simulink model "Experiment_0121_cs"  (R2019a)
settings: Solver=ode5  StartTime=0.0  StopTime=30  FixedStep=1/20  RelTol=1e-3
PreLoadFcn:
  | mbxruntime.callbacks.PreLoadFcn(bdroot);
PostLoadFcn:
  | mbxruntime.callbacks.PostLoadFcn(bdroot);
InitFcn:
  | mbxruntime.callbacks.InitFcn(bdroot);
StartFcn:
  | mbxruntime.callbacks.StartFcn(bdroot);
StopFcn:
  | mbxruntime.callbacks.StopFcn(bdroot);
model workspace (MAT data in the model file):
  mbox_table : struct (value not decoded)
  model_closed = 0
  sim_status = 0
undefined symbols (not defined in the file or in its folder): DiscIntNeverNeededParam, warningInitialVelocity, x0
libraries: simulink x37, PreScanSimulinkLibrary x16, simulink_extras x10, PreScanUsefulBlocks x1
(part 1 of 6)
CloseFcn:
  | mbxruntime.callbacks.CloseFcn(bdroot);
settings Model: Creator=PRESCAN  LastModifiedBy=HP
settings DataIOCC: LimitDataPoints=on  SaveFormat=Array  SignalLoggingSaveFormat=ModelDataLogs  ReturnWorkspaceOutputs=off
settings OptimizationCC: ExpressionDepthLimit=2147483647  InitFltsAndDblsToZero=on  LifeSpan=inf
settings DebuggingCC: SaveWithParameterizedLinksMsg=none  UnderspecifiedInitializationDetection=Classic  MergeDetectMultiDrivingBlocksExec=none  SignalResolutionControl=TryResolveAllWithWarning  MultiTaskDSMMsg=warning  MultiTaskCondExecSysMsg=none  FcnCallInpInsideContextMsg=warning  StateNameClashWarn=warning  SFUnexpectedBacktrackingDiag=warning  SFNoUnconditionalDefaultTransitionDiag=warning  SFExecutionAtInitializationDiag=none  ArithmeticOperatorsInVariantConditions=warning
settings HardwareCC: ProdBitPerPointer=32  ProdBitPerSizeT=32  ProdBitPerPtrDiffT=32  ProdLargestAtomicFloat=None  ProdIntDivRoundTo=Undefined  ProdEndianess=Unspecified  ProdWordSize=32  ProdHWDeviceType=32-bit Generic
settings ModelReferenceCC: UpdateModelReferenceTargets=IfOutOfDate  PropagateSignalLabelsOutOfModel=off
settings SFSimCC: SimUseLocalCustomCode=off  SimParseCustomCode=off
settings SFSimCC: SimCustomHeaderCode=|
  | #include "prescan.h"
  | #include "prescan_platform.h"
settings RTWCC: RTWUseLocalCustomCode=off
settings CodeAppCC: StateflowObjectComments=on
settings GRTTargetCC: TargetFcnLib=ansi_tfl_tmw.mat  TargetLangStandard=C89/C90 (ANSI)  GeneratePreprocessorConditionals=Disable all  CombineOutputUpdateFcns=off  GRTInterface=on
settings ConfigComp: CovMetricSettings=dw  CovHtmlReporting=on  CovSaveCumulativeToWorkspaceVar=on  CovSaveSingleToWorkspaceVar=on  CovExternalEMLEnable=off

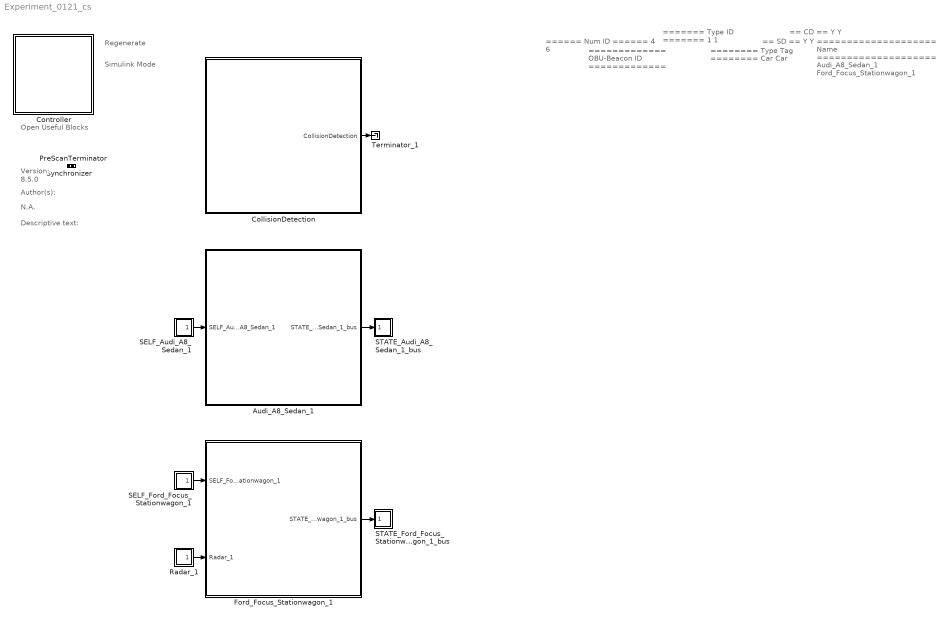
== system Experiment_0121_cs ==
  note: Regenerate
  note: Simulink Mode
  note: Open Useful Blocks
  note: 8.5.0
  note: Version:
  note: Author(s):
  note: N.A.
  note: Descriptive text:
  note: ======
      | Num ID
      | ======
      | 4
      | 6
  note: =============
      | OBU-Beacon ID
      | =============
  note: =======
      | Type ID
      | =======
      | 1
      | 1
  note: ========
      | Type Tag
      | ========
      | Car
      | Car
  note: ==
      | SD
      | ==
      | Y
      | Y
  note: ==
      | CD
      | ==
      | Y
      | Y
  note: ====================
      | Name
      | ====================
      | Audi_A8_Sedan_1
      | Ford_Focus_Stationwagon_1
  Audi_A8_Sedan_1 : Subsystem  Tag=WorldObjectSubSystem  InitFcn=UniqueId = '29';
      mask init:
      | modelPath = GenericModelHelper.getGenericModelFilePath('ModelDepo','Vehicles\Audi_A8\Audi_A8.pgmb','d771622804618130053427da08a6d484');imagePath = GenericModelHelper.getCompilationPicture(modelPath, 'Audi_A8_HighPoly.png');
      mask Display: image(imread(imagePath));color('white');text(0, 0, ' ID=4\n')
  CollisionDetection : Subsystem  Tag=sensor/CollisionDetection  Priority=3  LoadFcn=load('PrescanCollisionDetectionData.mat');load('PrescanCollisionDetectionMessage.mat')  mask(PreScan Source Block: CollisionDetection){}
      mask help: Collision Detection can be used to detect collisions between PreScan components. For Collision Detection the actual component shape is taken into account, so it is not a bounding box approach.
      settings: OpenFcn=open_system([gcb '/Sensor'],'mask')
      mask Help: eval('openHelp(811)')
      mask Display: image(imread('crash.jpg'))
  Controller : Subsystem  Description=35CC70460C0F6B9A74A5D35B42843DB509CCAA918CC068CE424F94149DBB7D73  Priority=-1  LoadFcn=load PreScanControllerData  mask(PreScan Simulation Controller){prescanversion='8.5.0', ModelReferencing=off, TimeStep=1/20, ControlMode=0, PreScanExecutionMode=on, ControllerCount=0, ControllerIndex=0, ControllerOptions=''}
      mask prompts: prescanversion "PreScan Version"; ModelReferencing "Use Model Referencing"; TimeStep "Upload Period [s]"; ControlMode "Control Mode"; PreScanExecutionMode "Execution Mode"; ControllerCount "Controller Count"; ControllerIndex "Controller Index"; ControllerOptions "Controller Options"
      mask help:
      | Please do not remove this block from the compilation sheet,
      | as it connects the model to the PreScan environment.
      mask init:
      | model = bdroot(gcb);
      | ExperimentFile = mbxruntime.findExperimentFile(model,true); %relative path
      | 
      | [d1, d2, d3, prescandata] = prescan_Settings();
      | ModelDepo = fullfile(prescandata,'ModelDepo'); 
      | 
      | RTmode = mbxruntime.getRTMode(model);
      | 
      | SimulationMode = get_param(bdroot,'SimulationMode');
      | if strcmp(SimulationMode, 'rapid-accelerator')
      |     SimulationMode = 'external';
      | end
      | TargetName = get_param(bdroot,'SystemTargetFile');
      settings: ModelCloseFcn=assignin('base',['model_closed_' bdroot],true);
      mask Help: eval('openHelp(812)')
      mask Display: image(imread('prescanlogo.ico'))
  Ford_Focus_Stationwagon_1 : Subsystem  Tag=WorldObjectSubSystem  InitFcn=UniqueId = '32';
      mask init:
      | modelPath = GenericModelHelper.getGenericModelFilePath('ModelDepo','Vehicles\Ford_Focus_Wagon\Ford_Focus_Wagon.pgmb','9f2f84850ce6f49365560c3439563633');imagePath = GenericModelHelper.getCompilationPicture(modelPath, 'Ford_Focus_Wagon_HighPoly.png');
      mask Display: image(imread(imagePath));color('white');text(0, 0, ' ID=6\n')
  PreScanTerminator : Subsystem  Tag=PreScanTerminator  Priority=999  LoadFcn=load PrescanTerminatorData  mask(PreScan Simulation Terminator){TimeStep=1/20}
      mask prompts: TimeStep "Upload Period [s]"
      mask help:
      | Please do not remove this block from the compilation sheet as it
      | connects the model to the PreScan environment.
      mask Help: eval('openHelp(812)')
      mask Display: image(imread('prescanlogo.ico'))
  Radar_1 : Subsystem  Tag=sensor/Radar  Priority=3  LoadFcn=load('PrescanScannerSensorData.mat');load('PrescanScannerSensorMessage.mat')  mask(PreScan Source Block: Radar Sensor){}
      mask help:
      | The Radar Sensor is a detailed sensor based on a physical radar
      | model that includes Antenna GAIN Maps (AGM) and atmospheric
      | attenuation.
      |
      | For more information, please click Help.
      settings: OpenFcn=open_system([gcb '/Sensor'],'mask')
      mask Help: eval('openHelp(1464)')
      mask Display: image(imread('Radar.png'))
  SELF_Audi_A8_Sedan_1 : Subsystem  Tag=sensor/SelfPort  Priority=3  LoadFcn=load('PreScanSelfSensorData.mat')  mask(PreScan Source Block: SELF){}
      mask help:
      | The SELF port shows (state) information of the actor itself. The outputs are position in the experiment's axis system and the GPS coordinates, and the object's absolute velocity and compass heading.
      |
      | For more information, please click Help.
      settings: OpenFcn=open_system([gcb '/Sensor'],'mask')
      mask Help: eval('openHelp(462)')
      mask Display: image(imread('GPS.png'))
  SELF_Ford_Focus_Stationwagon_1 : Subsystem  Tag=sensor/SelfPort  Priority=3  LoadFcn=load('PreScanSelfSensorData.mat')  mask(PreScan Source Block: SELF){}
      mask help:
      | The SELF port shows (state) information of the actor itself. The outputs are position in the experiment's axis system and the GPS coordinates, and the object's absolute velocity and compass heading.
      |
      | For more information, please click Help.
      settings: OpenFcn=open_system([gcb '/Sensor'],'mask')
      mask Help: eval('openHelp(462)')
      mask Display: image(imread('GPS.png'))
  STATE_Audi_A8_Sedan_1_bus : Subsystem  Tag=actuator/StatePort  Priority=0  LoadFcn=load('PreScanStateActuatorData.mat')  mask(PreScan Sink Block: State){}
      mask help:
      | The Actor State contains a vector signal of size (9x1), containing the following signals:
      |
      | -  Position    	(x,y,z)             	[m]
      | -  Velocity    	(vx,vy,vz)         	[m/s]
      | -  Angles       	(Roll, Pitch, Yaw)	[rad]
      |
      | The Actor state is defined in the global axis system.
      | The state is superponed on the Initial position defined in the GUI.
      |
      | For more information, please click Help.
      settings: OpenFcn=open_system([gcb '/Actuator'],'mask')
      mask Help: eval('openHelp(222)')
      mask Display: image(imread('State.png'))
  STATE_Ford_Focus_Stationwagon_1_bus : Subsystem  Tag=actuator/StatePort  Priority=0  LoadFcn=load('PreScanStateActuatorData.mat')  mask(PreScan Sink Block: State){}
      mask help:
      | The Actor State contains a vector signal of size (9x1), containing the following signals:
      |
      | -  Position    	(x,y,z)             	[m]
      | -  Velocity    	(vx,vy,vz)         	[m/s]
      | -  Angles       	(Roll, Pitch, Yaw)	[rad]
      |
      | The Actor state is defined in the global axis system.
      | The state is superponed on the Initial position defined in the GUI.
      |
      | For more information, please click Help.
      settings: OpenFcn=open_system([gcb '/Actuator'],'mask')
      mask Help: eval('openHelp(222)')
      mask Display: image(imread('State.png'))
  Synchronizer : Subsystem  Tag=PreScanSynchronizer  Priority=1  LoadFcn=load PrescanSynchronizeData  mask(PreScan Simulation Core Block){TimeStep=1/20}
      mask prompts: TimeStep "Timestep [s]"
      mask help:
      | Please do not remove this block from the PreScan compilation sheet,
      | as it contains essential configuration parameters for a PreScan simulation.
      settings: DeleteFcn=PreScanBlockDeleteFcn;
      mask Display: image(imread('prescanlogo.ico'))
  Terminator_1 : Terminator
  wires:
  Audi_A8_Sedan_1/1(STATE_Audi_A8_Sedan_1_bus) -> STATE_Audi_A8_Sedan_1_bus/1(STATE_Audi_A8_Sedan_1_bus)
  SELF_Audi_A8_Sedan_1/1(SELF_Audi_A8_Sedan_1) -> Audi_A8_Sedan_1/1(SELF_Audi_A8_Sedan_1)
  Ford_Focus_Stationwagon_1/1(STATE_Ford_Focus_Stationwagon_1_bus) -> STATE_Ford_Focus_Stationwagon_1_bus/1(STATE_Ford_Focus_Stationwagon_1_bus)
  SELF_Ford_Focus_Stationwagon_1/1(SELF_Ford_Focus_Stationwagon_1) -> Ford_Focus_Stationwagon_1/1(SELF_Ford_Focus_Stationwagon_1)
  Radar_1/1(Radar_1) -> Ford_Focus_Stationwagon_1/2(Radar_1)
  CollisionDetection/1(CollisionDetection) -> Terminator_1/1

== system Experiment_0121_cs/Audi_A8_Sedan_1 ==
  SELF_Audi_A8_Sedan_1 : Inport  Tag=inport/SelfPort  OutDataTypeStr=Bus: PRESCAN_SELFSENSORDATA  PortDimensions=1  SampleTime=1/20  BusOutputAsStruct=on
  Auto_Gear : Constant  Tag=AutoGear
  Dynamics_Simple : Subsystem  Tag=Simple_Vehicle_Dynamics  mask(PreScan Block: Simple Dynamics){Migrate=on, TimeStep=1/20, ComputationMode=Continuous_Time}
      mask prompts: Migrate "Migrate. During migration this block will be replaced by a newer one."; TimeStep "Auto assigned: Time Step [s]"; ComputationMode "Computation mode:"
      mask help:
      | The Simple Dynamics Model is selected in the GUI to simulate vehicle dynamics behavior.
      |
      | The Simple Dynamics Model is completely open to the user. The parameters of this model can be set in the Simple Dynamics dialog in the GUI.
      |
      | For more information, please click Help.
      mask init:
      | p = SimpleDyn_pars;
      settings: DeleteFcn=PreScanBlockDeleteFcn;
      mask Help: eval('openHelp(220)')
      mask Display:
      | image(imread('SimpleDyn.png'))
      | port_label('input', 1, '{\delta}_S_t_ _e_e_r [deg]','texmode','on')
      | port_label('input', 2, 'Throttle [%]')
      | port_label('input', 3, 'Brake Pres [bar]')
      | port_label('input', 4, 'V_0 [ms-1]','texmode','on')
      | port_label('input', 5, 'Auto=[0]/Manual=[1]')
      | port_label('input', 6, 'Auto_GearShift')
      | port_label('input', 7, 'Manual_GearShift')
      | port_label('output', 1, 'State')
      | port_label('output', 2, 'Vx [ms-1]')
      | port_label('output', 3, 'Perf Params')
  Ground_{1..6} (6 alike) : Ground
  SELF_Demux : Subsystem  Tag=demux/SelfPort  mask(PreScan Demux Block:){}
      mask help:
      | The SELF port shows (state) information of the actor itself. The outputs are position in the experiment's axis system and the GPS coordinates, and the object's absolute velocity and compass heading.
      |
      | For more information, please click Help.
      settings: DeleteFcn=PreScanBlockDeleteFcn;
      mask Help: eval('openHelp(462)')
      mask Display:
      | port_label('output',1,'x [m]')
      | port_label('output',2,'y [m]')
      | port_label('output',3,'z [m]','texmode','on')
      | port_label('output',4,'Rotx [deg]','texmode','on')
      | port_label('output',5,'Roty [deg]','texmode','on')
      | port_label('output',6,'Rotz [deg]','texmode','on')
      | port_label('output',7,'GPS lat [deg]','texmode','on')
      | port_label('output',8,'GPS long [deg]','texmode','on')
      | port_label('output',9,'GPS alt [m]','texmode','on')
      | port_label('output',10,'Velocity [m/s]')
      | port_label('output',11,'Heading [deg]')
      | port_label('output',12,'Yaw rate [deg/s]')
  STATE_Audi_A8_Sedan_1 : Subsystem  Tag=mux/StatePort  Priority=0  LoadFcn=load PrescanStateActuatorData  mask(PreScan Sink Block: State){x0=-266.0717, y0=106.8395, z0=0.55, Roll0=0, Pitch0=0, Yaw0=0, TimeStep=1/20}
      mask prompts: x0 "Ini x-position VEHICLE wrt GLOBAL axis system [m]"; y0 "Ini y-position VEHICLE wrt GLOBAL axis system [m]"; z0 "Ini z-position VEHICLE wrt GLOBAL axis system [m]"; Roll0 "Ini roll-angle BODY wrt VEHICLE axis system [deg]"; Pitch0 "Ini pitch-angle BODY wrt VEHICLE axis system [deg]"; Yaw0 "Ini yaw-angle VEHICLE wrt GLOBAL axis system [deg]"; TimeStep "Auto-Assigned: Upload Period [s]"
      mask help:
      | The Actor State contains a vector signal of size (9x1), containing the following signals:
      |
      | -  Position                  (x,y,z)                                     [m]
      | -  Velocity                  (vx,vy,vz)                               [m/s]
      | -  Angles                    (Roll, Pitch, Yaw)                   [rad]
      |
      | The Actor state is defined in the global axis system.
      | The state is superponed on the Initial position defined in the GUI.
      |
      | For more information, please click Help.
      settings: DeleteFcn=PreScanBlockDeleteFcn;
      mask Help: eval('openHelp(222)')
      mask Display: image(imread('State.png'))
  STATE_Audi_A8_Sedan_1_rc : RateTransition  Tag=mux_rc/StatePort  OutPortSampleTimeOpt=Inherit
  Terminator_{1..15} (15 alike) : Terminator
  Trajectories : Subsystem  Tag=Trajectories  mask(PreScan Source Block: Trajectories){}
      mask help:
      | The Trajectory block contains the trajectories defined in the PreScan Experiment Editor. The output of the trajectory block is the (vehicle) State.
      |
      | For more information, please click Help.
      settings: DeleteFcn=PreScanBlockDeleteFcn;
      mask Help: eval('openHelp(312)')
      mask Display: image(imread('Trajectory.png'));
  STATE_Audi_A8_Sedan_1_bus : Outport  Tag=outport/StatePort  OutDataTypeStr=Bus: PRESCAN_STATEACTUATORDATA  PortDimensions=1  SampleTime=1/20
  wires:
  STATE_Audi_A8_Sedan_1_rc/1 -> STATE_Audi_A8_Sedan_1_bus/1
  STATE_Audi_A8_Sedan_1/1(StateBus) -> STATE_Audi_A8_Sedan_1_rc/1
  SELF_Audi_A8_Sedan_1/1 -> SELF_Demux/1(SELF)
  Auto_Gear/1 -> Dynamics_Simple/6(Auto_GearShift)
  Dynamics_Simple/1(State) -> STATE_Audi_A8_Sedan_1/1(State)
  Ground_1/1 -> Dynamics_Simple/1(DeltaSteer_[deg])
  Ground_2/1 -> Dynamics_Simple/2(Throttle)
  Ground_3/1 -> Dynamics_Simple/3(Brake)
  Ground_4/1 -> Dynamics_Simple/4(Initial_Vx_[ms-1])
  Ground_5/1 -> Dynamics_Simple/5(AutoManual_OnOff)
  Ground_6/1 -> Dynamics_Simple/7(Manual_GearShift)
  Dynamics_Simple/2(Vx [m s-1]) -> Terminator_1/1
  Dynamics_Simple/3(Perf_Params) -> Terminator_2/1
  SELF_Demux/1(x [m]) -> Terminator_3/1
  SELF_Demux/2(y [m]) -> Terminator_4/1
  SELF_Demux/3(z [m]) -> Terminator_5/1
  SELF_Demux/4(rotx [deg]) -> Terminator_6/1
  SELF_Demux/5(roty [deg]) -> Terminator_7/1
  SELF_Demux/6(rotz [deg]) -> Terminator_8/1
  SELF_Demux/7(GPS lat [deg]) -> Terminator_9/1
  SELF_Demux/8(GPS long [deg]) -> Terminator_10/1
  SELF_Demux/9(GPS alt [m]) -> Terminator_11/1
  SELF_Demux/10(velocity [m/s]) -> Terminator_12/1
  SELF_Demux/11(heading [deg]) -> Terminator_13/1
  SELF_Demux/12(yaw rate [deg/s]) -> Terminator_14/1
  Trajectories/1(State) -> Terminator_15/1

== system Experiment_0121_cs/CollisionDetection ==
  Sensor : S-Function  FunctionName=sfun_CollisionDetection  Parameters=detectableCollisions, timestep  SFunctionDeploymentMode=off  EnableBusSupport=off  mask(PreScan Source Block: CollisionDetection){detectableCollisions=5, timestep=1/20}
      mask prompts: detectableCollisions "Max detectable collisions:"; timestep "MATLAB timestep:"
      mask help: Collision Detection can be used to detect collisions between PreScan components. For Collision Detection the actual component shape is taken into account, so it is not a bounding box approach.
      mask Help: eval('openHelp(811)')
      mask Display: image(imread('crash.jpg'))
  CollisionDetection : Outport  Tag=outport/CollisionDetection  OutDataTypeStr=Bus: PRESCAN_COLLISIONDETECTION_MESSAGE  PortDimensions=5  SampleTime=1/20
  wires:
  Sensor/1 -> CollisionDetection/1

== system Experiment_0121_cs/Controller ==
  Terminator : Terminator
  sfun_Controller : S-Function  FunctionName=sfun_Controller  Parameters=SParameter1, SParameter2, SParameter3, SParameter4, SParameter5, SParameter6, SParameter7, SParameter8, SParameter9, SParameter10, SampleTime  SFunctionDeploymentMode=off  EnableBusSupport=off  mask(Legacy Function){SFunctionSpec=void prescan_outputFcn(void** work1, PRESCAN_CONTROLLERDATA y1[1]), SParameter1=uint8([ExperimentFile 0]), SParameter2=uint8([ModelDepo 0]), SParameter3=uint8([ControllerOptions 0]), SParameter4=RTmode, SParameter5=PreScanExecutionMode, SParameter6=ControlMode, SParameter7=ControllerCount, SParameter8=ControllerIndex, SParameter9=uint8([SimulationMode 0]), SParameter10=uint8([TargetName 0]), SampleTime=TimeStep, ShowSpec=on}
      mask prompts: SParameter1 "P1:"; SParameter2 "P2:"; SParameter3 "P3:"; SParameter4 "P4:"; SParameter5 "P5:"; SParameter6 "P6:"; SParameter7 "P7:"; SParameter8 "P8:"; SParameter9 "P9:"; SParameter10 "P10:"; SampleTime "Sample time (-1 for inherited):"; ShowSpec "Display function specification"
      mask help:
      | This block allows you to call the legacy functions specified by the following Legacy Code Tool definition:
      | def.SFunctionName = 'sfun_Controller';
      | def.OutputFcnSpec = 'void prescan_outputFcn(void** work1, PRESCAN_CONTROLLERDATA y1[1])';
      | def.StartFcnSpec = 'void prescan_startFcn(void ** work1, uint8 p1[], uint8 p2[], uint8 p3[], double p4, double p5, double p6, double p7, double p8, uint8 p9[], uint8 p10[])';
      | def.TerminateFcnSpec = 'void prescan_terminateFcn(void** work1)';
      | def.HeaderFiles = {'prescan_controller_data.h', 'prescan_SFunLibrary.h', 'prescan_CreateLogHandler.h', 'prescan_CreateErrorHandler.h', 'prescan_modify.h', 'ModuleDLL.h'};
      | def.SourceFiles = {'prescan_MexLogHandler.c', 'prescan_SimStructErrorHandler.c', 'prescan_LogHandler.c', 'prescan_ErrorHandler.c', 'prescan_Modify.c'};
      | def.HostLibFiles = {'sensorinterfaced.lib'};
      | def.TargetLibFiles = {'sensorinterfaced.so'};
      | def.IncPaths = {'.', 'C:\projects\prescan\rt_vislibrary\vis\..\pimp\include\sensors\InterfaceRTW'};
      | def.SrcPaths = {'C:\projects\prescan\rt_vislibrary\vis\..\pimp\include\sensors\InterfaceRTW', 'C:\projects\prescan\rt_vislibrary\vis\..\pimp\include\sensors\InterfaceRTW\ccurrt'};
      | def.LibPaths = {'C:\\projects\\prescan\\vislibrary_build\lib'};
      | def.SampleTime = 'parameterized';
      mask Help: <p>This block was generated automatically by the Legacy Code Tool. For detailed help on this tool, call<a href="matlab:legacy_code('help')"> legacy_code('help')</a>.</p>
      mask Callback ShowSpec:
      | if strcmp(get_param(gcbh, 'ShowSpec'), 'on')
      |   set_param(gcbh, 'MaskDisplay', sprintf('fprintf(''%s'');', get_param(gcbh, 'SFunctionSpec')));
      | else
      |   set_param(gcbh, 'MaskDisplay', sprintf('fprintf(''%s'');', get_param(gcbh, 'FunctionName')));
      | end
      mask Display: fprintf('void prescan_outputFcn(void** work1, PRESCAN_CONTROLLERDATA y1[1])');
  wires:
  sfun_Controller/1 -> Terminator/1

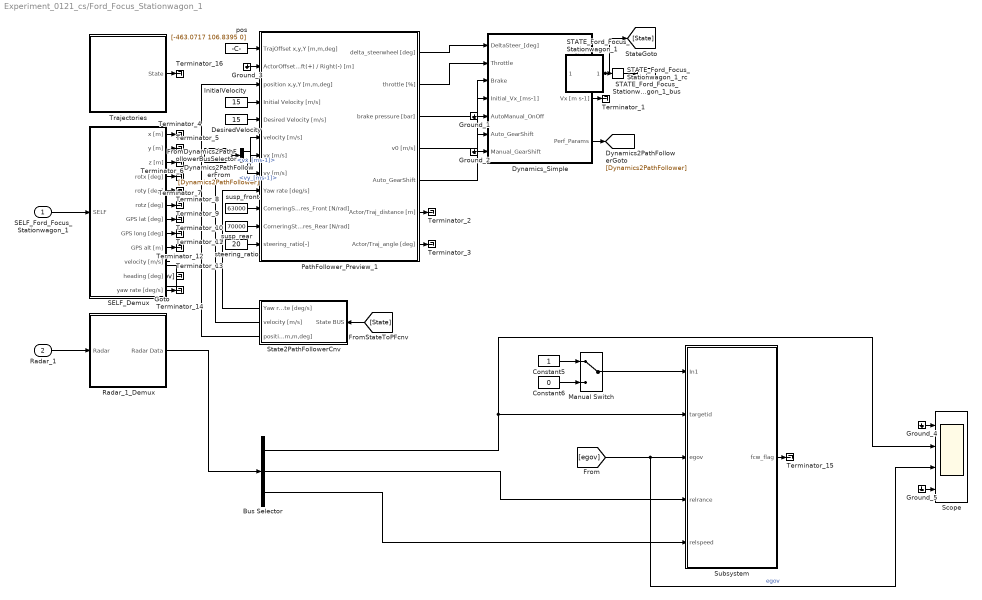
== system Experiment_0121_cs/Ford_Focus_Stationwagon_1 ==
  SELF_Ford_Focus_Stationwagon_1 : Inport  Tag=inport/SelfPort  OutDataTypeStr=Bus: PRESCAN_SELFSENSORDATA  PortDimensions=1  SampleTime=1/20  BusOutputAsStruct=on
  Radar_1 : Inport  Tag=inport/Radar  Port=2  OutDataTypeStr=Bus: PRESCAN_SCANNERSENSOR_MESSAGE  PortDimensions=7  SampleTime=1/20  BusOutputAsStruct=on
  Bus Selector : BusSelector  OutputSignals=TargetID[-],Range[m],DopplerVelocityX[ms-1]
  Constant5 : Constant
  Constant6 : Constant  Value=0
  DesiredVelocity : Constant  Tag=DesiredVelocity  Value=15
  Dynamics_Simple : Subsystem  Tag=Simple_Vehicle_Dynamics  mask(PreScan Block: Simple Dynamics){Migrate=on, TimeStep=1/20, ComputationMode=Continuous_Time}
      mask prompts: Migrate "Migrate. During migration this block will be replaced by a newer one."; TimeStep "Auto assigned: Time Step [s]"; ComputationMode "Computation mode:"
      mask help:
      | The Simple Dynamics Model is selected in the GUI to simulate vehicle dynamics behavior.
      |
      | The Simple Dynamics Model is completely open to the user. The parameters of this model can be set in the Simple Dynamics dialog in the GUI.
      |
      | For more information, please click Help.
      mask init:
      | p = SimpleDyn_pars;
      settings: DeleteFcn=PreScanBlockDeleteFcn;
      mask Help: eval('openHelp(220)')
      mask Display:
      | image(imread('SimpleDyn.png'))
      | port_label('input', 1, '{\delta}_S_t_ _e_e_r [deg]','texmode','on')
      | port_label('input', 2, 'Throttle [%]')
      | port_label('input', 3, 'Brake Pres [bar]')
      | port_label('input', 4, 'V_0 [ms-1]','texmode','on')
      | port_label('input', 5, 'Auto=[0]/Manual=[1]')
      | port_label('input', 6, 'Auto_GearShift')
      | port_label('input', 7, 'Manual_GearShift')
      | port_label('output', 1, 'State')
      | port_label('output', 2, 'Vx [ms-1]')
      | port_label('output', 3, 'Perf Params')
  FromDynamics2PathFollowerBusSelector : BusSelector  OutputSignals=vx_[ms-1],vy_[ms-1]
  Ground_{1..5} (5 alike) : Ground
  InitialVelocity : Constant  Tag=InitialVelocity  Value=15
  Manual Switch : ManualSwitch
  PathFollower_Preview_1 : Subsystem  Tag=PathFollower_Preview  mask(PreScan Block: Path Follower with Preview){Migrate=on, LongCtrl_P=20, LongCtrl_I=0.3, LongCtrl_D=3.065, LongCtrl_AWU=1, LongCtrlDefault_P=20, LongCtrlDefault_I=0.3, LongCtrlDefault_D=3.065, LongCtrlDefault_AWU=1, FileName='Trajectory_2.mat', mass=1471, Jzz=1500, length_a=2.65 - 1.45, length_l=2.65, Angle_Max_SteeringWheel=500, PreviewTime=1, DelayTime=0.1, LowSpeedLimit=20, MaxSteeringRate=1200, CSSampleTime=1/20, PFIntegrationFrequency=20}
      mask prompts: Migrate "Migrate. During migration this block will be replaced by a newer one."; LongCtrl_P "Longitudinal Controller P"; LongCtrl_I "Longitudinal Controller I"; LongCtrl_D "Longitudinal Controller D"; LongCtrl_AWU "Longitudinal Controller AWU"; FileName "Trajectory Name"; mass "Mass vehicle total [kg]"; Jzz "Inertia vehicle around yaw axis [kg m2]"; length_a "Distance between COG and front axle [m]"; length_l "Length of wheelbase [m]"; Angle_Max_SteeringWheel "Maximum steering wheel angle [deg]"; PreviewTime "Preview time [s]"; DelayTime "Delay time [s]"; LowSpeedLimit "Low-speed limit [km/h]"; MaxSteeringRate "Maximum steering wheel angle rate [deg/s]"; CSSampleTime "Compilation Sheet sample time [s]"; PFIntegrationFrequency "Lateral controller frequency [Hz]"
      mask help:
      | The Path Follower Model is selected in the GUI to simulate driver behavior.
      |
      | For more information, please click Help.
      mask init:
      | load(['trajectories/',eval(FileName)])
      | traject=trajectory';
      | 
      | Traj_x=traject(:,2);
      | Traj_y=traject(:,3);
      | Traj_t=traject(2,1);
      | Traj_v=sqrt(traject(:,8).^2+traject(:,9).^2+traject(:,10).^2);
      | 
      | RefreshCounter = max(floor((1/CSSampleTime) / (PFIntegrationFrequency)), 1); %Compilation sheet frequency/path follower frequency
      | 
      | blockPath = gcb;
      | 
      | clear traject;
      mask Help: eval('openHelp(233)')
      mask DialogControl Container12 Prompt: Controller Parameters
      mask DialogControl Control2 Prompt: Reset PID parameters
      mask DialogControl Control2 Callback:
      | LongCtrlDefault_P = get_param(gcb,'LongCtrlDefault_P');
      | set_param(gcb,'LongCtrl_P',LongCtrlDefault_P);
      | 
      | LongCtrlDefault_I = get_param(gcb,'LongCtrlDefault_I');
      | set_param(gcb,'LongCtrl_I',LongCtrlDefault_I);
      | 
      | LongCtrlDefault_D = get_param(gcb,'LongCtrlDefault_D');
      | set_param(gcb,'LongCtrl_D',LongCtrlDefault_D);
      | 
      | LongCtrlDefault_AWU = get_param(gcb,'LongCtrlDefault_AWU');
      | set_param(gcb,'LongCtrl_AWU',LongCtrlDefault_AWU);
      mask DialogControl Container10 Prompt: System Parameters
  Radar_1_Demux : Subsystem  Tag=demux/Radar  TreatAsAtomicUnit=on  mask(PreScan Demux Block: Radar){MAXMESSAGES=7}
      mask prompts: MAXMESSAGES "Number of Objects"
      mask help:
      | The Radar Sensor is a detailed sensor based on a physical radar
      | model that includes Antenna GAIN Maps (AGM) and atmospheric
      | attenuation.
      |
      | For more information, please click Help.
      mask Help: eval('openHelp(1464)')
      mask Display:
      | port_label('input',1,'Radar')
      | port_label('output',1,'Radar Data')
  SELF_Demux : Subsystem  Tag=demux/SelfPort  mask(PreScan Demux Block:){}
      mask help:
      | The SELF port shows (state) information of the actor itself. The outputs are position in the experiment's axis system and the GPS coordinates, and the object's absolute velocity and compass heading.
      |
      | For more information, please click Help.
      settings: DeleteFcn=PreScanBlockDeleteFcn;
      mask Help: eval('openHelp(462)')
      mask Display:
      | port_label('output',1,'x [m]')
      | port_label('output',2,'y [m]')
      | port_label('output',3,'z [m]','texmode','on')
      | port_label('output',4,'Rotx [deg]','texmode','on')
      | port_label('output',5,'Roty [deg]','texmode','on')
      | port_label('output',6,'Rotz [deg]','texmode','on')
      | port_label('output',7,'GPS lat [deg]','texmode','on')
      | port_label('output',8,'GPS long [deg]','texmode','on')
      | port_label('output',9,'GPS alt [m]','texmode','on')
      | port_label('output',10,'Velocity [m/s]')
      | port_label('output',11,'Heading [deg]')
      | port_label('output',12,'Yaw rate [deg/s]')
  STATE_Ford_Focus_Stationwagon_1 : Subsystem  Tag=mux/StatePort  Priority=0  LoadFcn=load PrescanStateActuatorData  mask(PreScan Sink Block: State){x0=-463.0717, y0=106.8395, z0=0.5, Roll0=0, Pitch0=0, Yaw0=0, TimeStep=1/20}
      mask prompts: x0 "Ini x-position VEHICLE wrt GLOBAL axis system [m]"; y0 "Ini y-position VEHICLE wrt GLOBAL axis system [m]"; z0 "Ini z-position VEHICLE wrt GLOBAL axis system [m]"; Roll0 "Ini roll-angle BODY wrt VEHICLE axis system [deg]"; Pitch0 "Ini pitch-angle BODY wrt VEHICLE axis system [deg]"; Yaw0 "Ini yaw-angle VEHICLE wrt GLOBAL axis system [deg]"; TimeStep "Auto-Assigned: Upload Period [s]"
      mask help:
      | The Actor State contains a vector signal of size (9x1), containing the following signals:
      |
      | -  Position                  (x,y,z)                                     [m]
      | -  Velocity                  (vx,vy,vz)                               [m/s]
      | -  Angles                    (Roll, Pitch, Yaw)                   [rad]
      |
      | The Actor state is defined in the global axis system.
      | The state is superponed on the Initial position defined in the GUI.
      |
      | For more information, please click Help.
      settings: DeleteFcn=PreScanBlockDeleteFcn;
      mask Help: eval('openHelp(222)')
      mask Display: image(imread('State.png'))
  STATE_Ford_Focus_Stationwagon_1_rc : RateTransition  Tag=mux_rc/StatePort  OutPortSampleTimeOpt=Inherit
  Scope : Scope  NumInputPorts=4
  State2PathFollowerCnv : Subsystem  Tag=State2PFConnection/cnv
  Subsystem : Subsystem
  Terminator_{1..16} (16 alike) : Terminator
  Trajectories : Subsystem  Tag=Trajectories  mask(PreScan Source Block: Trajectories){}
      mask help:
      | The Trajectory block contains the trajectories defined in the PreScan Experiment Editor. The output of the trajectory block is the (vehicle) State.
      |
      | For more information, please click Help.
      settings: DeleteFcn=PreScanBlockDeleteFcn;
      mask Help: eval('openHelp(312)')
      mask Display: image(imread('Trajectory.png'));
  pos : Constant  Tag=pos  Value=[-463.0717 106.8395 0]
  steering_ratio : Constant  Tag=steering_ratio  Value=20
  susp_front : Constant  Tag=susp_front  Value=63000
  susp_rear : Constant  Tag=susp_rear  Value=70000
  STATE_Ford_Focus_Stationwagon_1_bus : Outport  Tag=outport/StatePort  OutDataTypeStr=Bus: PRESCAN_STATEACTUATORDATA  PortDimensions=1  SampleTime=1/20
  wires:
  Bus Selector/1 -> Subsystem/2(targetid), Scope/2
  Manual Switch/1 -> Subsystem/1(In1)
  Constant5/1 -> Manual Switch/1
  Constant6/1 -> Manual Switch/2
  [egov] -> Subsystem/3(egov), Scope/3  "egov"
  Bus Selector/2 -> Subsystem/4(relrance)
  Bus Selector/3 -> Subsystem/5(relspeed)
  Radar_1_Demux/1(Radar Data) -> Bus Selector/1
  SELF_Demux/10(velocity [m/s]) -> [egov]
  STATE_Ford_Focus_Stationwagon_1_rc/1 -> STATE_Ford_Focus_Stationwagon_1_bus/1
  STATE_Ford_Focus_Stationwagon_1/1(StateBus) -> STATE_Ford_Focus_Stationwagon_1_rc/1, [State]
  SELF_Ford_Focus_Stationwagon_1/1 -> SELF_Demux/1(SELF)
  Radar_1/1 -> Radar_1_Demux/1(Radar)
  pos/1 -> PathFollower_Preview_1/1(TrajOffset x,y,Y [m,m,deg])
  susp_front/1 -> PathFollower_Preview_1/10(CorneringStiffness_Tyres_Front [N/rad])
  susp_rear/1 -> PathFollower_Preview_1/11(CorneringStiffness_Tyres_Rear [N/rad])
  steering_ratio/1 -> PathFollower_Preview_1/12(steering_ratio[-])
  InitialVelocity/1 -> PathFollower_Preview_1/4(Initial Velocity [m/s])
  DesiredVelocity/1 -> PathFollower_Preview_1/5(Desired Velocity [m/s])
  [State] -> State2PathFollowerCnv/1(State BUS)
  State2PathFollowerCnv/1(Yaw rate [deg/s]) -> PathFollower_Preview_1/9(Yaw rate [deg/s])
  State2PathFollowerCnv/2(velocity [m/s]) -> PathFollower_Preview_1/6(velocity [m/s])
  State2PathFollowerCnv/3(position x,y,Y [m,m,deg]) -> PathFollower_Preview_1/3(position x,y,Y [m,m,deg])
  PathFollower_Preview_1/1(delta_steerwheel [deg]) -> Dynamics_Simple/1(DeltaSteer_[deg])
  PathFollower_Preview_1/2(throttle [%]) -> Dynamics_Simple/2(Throttle)
  PathFollower_Preview_1/3(brake pressure [bar]) -> Dynamics_Simple/3(Brake)
  PathFollower_Preview_1/4(v0 [m/s]) -> Dynamics_Simple/4(Initial_Vx_[ms-1])
  PathFollower_Preview_1/5(Auto_GearShift) -> Dynamics_Simple/6(Auto_GearShift)
  Dynamics_Simple/3(Perf_Params) -> [Dynamics2PathFollower]
  FromDynamics2PathFollowerBusSelector/1 -> PathFollower_Preview_1/7(vx [m/s])  "<vx_[ms-1]>"
  FromDynamics2PathFollowerBusSelector/2 -> PathFollower_Preview_1/8(vy [m/s])  "<vy_[ms-1]>"
  [Dynamics2PathFollower] -> FromDynamics2PathFollowerBusSelector/1
  Dynamics_Simple/1(State) -> STATE_Ford_Focus_Stationwagon_1/1(State)
  Ground_1/1 -> Dynamics_Simple/5(AutoManual_OnOff)
  Ground_2/1 -> Dynamics_Simple/7(Manual_GearShift)
  Dynamics_Simple/2(Vx [m s-1]) -> Terminator_1/1
  Ground_3/1 -> PathFollower_Preview_1/2(ActorOffset_Left(+) / Right(-) [m])
  PathFollower_Preview_1/6(Actor/Traj_distance [m]) -> Terminator_2/1
  PathFollower_Preview_1/7(Actor/Traj_angle [deg]) -> Terminator_3/1
  SELF_Demux/1(x [m]) -> Terminator_4/1
  SELF_Demux/2(y [m]) -> Terminator_5/1
  SELF_Demux/3(z [m]) -> Terminator_6/1
  SELF_Demux/4(rotx [deg]) -> Terminator_7/1
  SELF_Demux/5(roty [deg]) -> Terminator_8/1
  SELF_Demux/6(rotz [deg]) -> Terminator_9/1
  SELF_Demux/7(GPS lat [deg]) -> Terminator_10/1
  SELF_Demux/8(GPS long [deg]) -> Terminator_11/1
  SELF_Demux/9(GPS alt [m]) -> Terminator_12/1
  SELF_Demux/11(heading [deg]) -> Terminator_13/1
  SELF_Demux/12(yaw rate [deg/s]) -> Terminator_14/1
  Ground_4/1 -> Scope/1
  Ground_5/1 -> Scope/4
  Subsystem/1(fcw_flag) -> Terminator_15/1
  Trajectories/1(State) -> Terminator_16/1

== system Experiment_0121_cs/PreScanTerminator ==
  Terminator : Terminator
  sfun_Terminator : S-Function  FunctionName=sfun_Terminator  Parameters=SampleTime  SFunctionDeploymentMode=off  EnableBusSupport=off  mask(Legacy Function){SFunctionSpec=void prescan_terminator_outputFcn(void ** work1, PRESCAN_TERMINATORDATA y1[1]), SampleTime=TimeStep, ShowSpec=on}
      mask prompts: SampleTime "Sample time (-1 for inherited):"; ShowSpec "Display function specification"
      mask help:
      | This block allows you to call the legacy functions specified by the following Legacy Code Tool definition:
      | def.SFunctionName = 'sfun_Terminator';
      | def.OutputFcnSpec = 'void prescan_terminator_outputFcn(void ** work1, PRESCAN_TERMINATORDATA y1[1])';
      | def.StartFcnSpec = 'void prescan_terminator_startFcn(void ** work1)';
      | def.TerminateFcnSpec = 'void prescan_terminator_terminateFcn(void ** work1)';
      | def.HeaderFiles = {'prescan_terminator_data.h'};
      | def.HostLibFiles = {'sensorinterfaced.lib'};
      | def.IncPaths = {'src', 'C:\prescandev\vislibrary\vis\..\pimp\include\sensors\InterfaceRTW'};
      | def.SrcPaths = {'src'};
      | def.LibPaths = {'C:\\prescandev\\vislibrary_build\lib'};
      | def.SampleTime = 'parameterized';
      | def.Options.language = 'C';
      mask Help: <p>This block was generated automatically by the Legacy Code Tool. For detailed help on this tool, call<a href="matlab:legacy_code('help')"> legacy_code('help')</a>.</p>
      mask Callback ShowSpec:
      | if strcmp(get_param(gcbh, 'ShowSpec'), 'on')
      |   set_param(gcbh, 'MaskDisplay', sprintf('fprintf(''%s'');', get_param(gcbh, 'SFunctionSpec')));
      | else
      |   set_param(gcbh, 'MaskDisplay', sprintf('fprintf(''%s'');', get_param(gcbh, 'FunctionName')));
      | end
      mask Display: fprintf('void prescan_terminator_outputFcn(void ** work1, PRESCAN_TERMINATORDATA y1[1])');
  wires:
  sfun_Terminator/1 -> Terminator/1

== system Experiment_0121_cs/Radar_1 ==
  Sensor : S-Function  FunctionName=sfun_Radar  Parameters=sensorID, detectableObjects, timestep  SFunctionDeploymentMode=off  EnableBusSupport=off  mask(PreScan Source Block: Radar Sensor){sensorID=36, detectableObjects=7, timestep=1/20}
      mask prompts: sensorID "Sensor ID"; detectableObjects "Max detectable objects:"; timestep "MATLAB timestep:"
      mask help:
      | The Radar Sensor is a detailed sensor based on a physical radar
      | model that includes Antenna GAIN Maps (AGM) and atmospheric
      | attenuation.
      |
      | For more information, please click Help.
      mask Help: eval('openHelp(1464)')
      mask Display: image(imread('Radar.png'))
  Radar_1 : Outport  Tag=outport/Radar  OutDataTypeStr=Bus: PRESCAN_SCANNERSENSOR_MESSAGE  PortDimensions=7  SampleTime=1/20
  wires:
  Sensor/1 -> Radar_1/1

== system Experiment_0121_cs/SELF_Audi_A8_Sedan_1 ==
  Sensor : S-Function  FunctionName=sfun_SelfSensor  Parameters=UniqueID, TimeStep  SFunctionDeploymentMode=off  EnableBusSupport=off  mask(PreScan Source Block: SELF){UniqueID=29, TimeStep=1/20}
      mask prompts: UniqueID "Auto-Assigned: Unique ID"; TimeStep "Auto-Assigned: Upload Period [s]"
      mask help:
      | The SELF port shows (state) information of the actor itself. The outputs are position in the experiment's axis system and the GPS coordinates, and the object's absolute velocity and compass heading.
      |
      | For more information, please click Help.
      mask Help: eval('openHelp(462)')
      mask Display: image(imread('GPS.png'))
  SELF_Audi_A8_Sedan_1 : Outport  Tag=outport/SelfPort  OutDataTypeStr=Bus: PRESCAN_SELFSENSORDATA  PortDimensions=1  SampleTime=1/20
  wires:
  Sensor/1 -> SELF_Audi_A8_Sedan_1/1

== system Experiment_0121_cs/SELF_Ford_Focus_Stationwagon_1 ==
  Sensor : S-Function  FunctionName=sfun_SelfSensor  Parameters=UniqueID, TimeStep  SFunctionDeploymentMode=off  EnableBusSupport=off  mask(PreScan Source Block: SELF){UniqueID=32, TimeStep=1/20}
      mask prompts: UniqueID "Auto-Assigned: Unique ID"; TimeStep "Auto-Assigned: Upload Period [s]"
      mask help:
      | The SELF port shows (state) information of the actor itself. The outputs are position in the experiment's axis system and the GPS coordinates, and the object's absolute velocity and compass heading.
      |
      | For more information, please click Help.
      mask Help: eval('openHelp(462)')
      mask Display: image(imread('GPS.png'))
  SELF_Ford_Focus_Stationwagon_1 : Outport  Tag=outport/SelfPort  OutDataTypeStr=Bus: PRESCAN_SELFSENSORDATA  PortDimensions=1  SampleTime=1/20
  wires:
  Sensor/1 -> SELF_Ford_Focus_Stationwagon_1/1

== system Experiment_0121_cs/STATE_Audi_A8_Sedan_1_bus ==
  STATE_Audi_A8_Sedan_1_bus : Inport  Tag=inport/StatePort  OutDataTypeStr=Bus: PRESCAN_STATEACTUATORDATA  PortDimensions=1  SampleTime=1/20  BusOutputAsStruct=on
  Actuator : S-Function  FunctionName=sfun_StateActuator  Parameters=UniqueID, TimeStep  SFunctionDeploymentMode=off  EnableBusSupport=off  mask(PreScan Sink Block: State){UniqueID=29, TimeStep=1/20}
      mask prompts: UniqueID "Auto-Assigned: Unique ID"; TimeStep "Auto-Assigned: Upload Period [s]"
      mask help:
      | The Actor State contains a vector signal of size (9x1), containing the following signals:
      |
      | -  Position    	(x,y,z)             	[m]
      | -  Velocity    	(vx,vy,vz)         	[m/s]
      | -  Angles       	(Roll, Pitch, Yaw)	[rad]
      |
      | The Actor state is defined in the global axis system.
      | The state is superponed on the Initial position defined in the GUI.
      |
      | For more information, please click Help.
      mask Help: eval('openHelp(222)')
      mask Display: image(imread('State.png'))
  wires:
  STATE_Audi_A8_Sedan_1_bus/1 -> Actuator/1

== system Experiment_0121_cs/STATE_Ford_Focus_Stationwagon_1_bus ==
  STATE_Ford_Focus_Stationwagon_1_bus : Inport  Tag=inport/StatePort  OutDataTypeStr=Bus: PRESCAN_STATEACTUATORDATA  PortDimensions=1  SampleTime=1/20  BusOutputAsStruct=on
  Actuator : S-Function  FunctionName=sfun_StateActuator  Parameters=UniqueID, TimeStep  SFunctionDeploymentMode=off  EnableBusSupport=off  mask(PreScan Sink Block: State){UniqueID=32, TimeStep=1/20}
      mask prompts: UniqueID "Auto-Assigned: Unique ID"; TimeStep "Auto-Assigned: Upload Period [s]"
      mask help:
      | The Actor State contains a vector signal of size (9x1), containing the following signals:
      |
      | -  Position    	(x,y,z)             	[m]
      | -  Velocity    	(vx,vy,vz)         	[m/s]
      | -  Angles       	(Roll, Pitch, Yaw)	[rad]
      |
      | The Actor state is defined in the global axis system.
      | The state is superponed on the Initial position defined in the GUI.
      |
      | For more information, please click Help.
      mask Help: eval('openHelp(222)')
      mask Display: image(imread('State.png'))
  wires:
  STATE_Ford_Focus_Stationwagon_1_bus/1 -> Actuator/1

== system Experiment_0121_cs/Synchronizer ==
  Bus Selector1 : BusSelector  OutputSignals=FederateStopped
  Stop Simulation : Stop
  sfun_Synchronizer : S-Function  FunctionName=sfun_Synchronizer  Parameters=SampleTime  SFunctionDeploymentMode=off  EnableBusSupport=off  mask(Legacy Function){SFunctionSpec=void prescan_synchronizer_outputFcn(void ** work1, PRESCAN_SYNCHRONIZEDATA y1[1]), SampleTime=TimeStep, ShowSpec=on}
      mask prompts: SampleTime "Sample time (-1 for inherited):"; ShowSpec "Display function specification"
      mask help:
      | This block allows you to call the legacy functions specified by the following Legacy Code Tool definition:
      | def.SFunctionName = 'sfun_Synchronizer';
      | def.OutputFcnSpec = 'void prescan_synchronizer_outputFcn(void ** work1, PRESCAN_SYNCHRONIZEDATA y1[1])';
      | def.StartFcnSpec = 'void prescan_synchronizer_startFcn(void ** work1)';
      | def.TerminateFcnSpec = 'void prescan_synchronizer_terminateFcn(void ** work1)';
      | def.HeaderFiles = {'prescan_synchronizer_data.h'};
      | def.HostLibFiles = {'sensorinterfaced.lib'};
      | def.IncPaths = {'src', 'C:\prescandev\vislibrary\vis\..\pimp\include\sensors\InterfaceRTW'};
      | def.SrcPaths = {'src'};
      | def.LibPaths = {'C:\\prescandev\\vislibrary_build\lib'};
      | def.SampleTime = 'parameterized';
      | def.Options.language = 'C';
      mask Help: <p>This block was generated automatically by the Legacy Code Tool. For detailed help on this tool, call<a href="matlab:legacy_code('help')"> legacy_code('help')</a>.</p>
      mask Callback ShowSpec:
      | if strcmp(get_param(gcbh, 'ShowSpec'), 'on')
      |   set_param(gcbh, 'MaskDisplay', sprintf('fprintf(''%s'');', get_param(gcbh, 'SFunctionSpec')));
      | else
      |   set_param(gcbh, 'MaskDisplay', sprintf('fprintf(''%s'');', get_param(gcbh, 'FunctionName')));
      | end
      mask Display: fprintf('void prescan_synchronizer_outputFcn(void ** work1, PRESCAN_SYNCHRONIZEDATA y1[1])');
  wires:
  Bus Selector1/1 -> Stop Simulation/1  "<FederateStopped>"
  sfun_Synchronizer/1 -> Bus Selector1/1

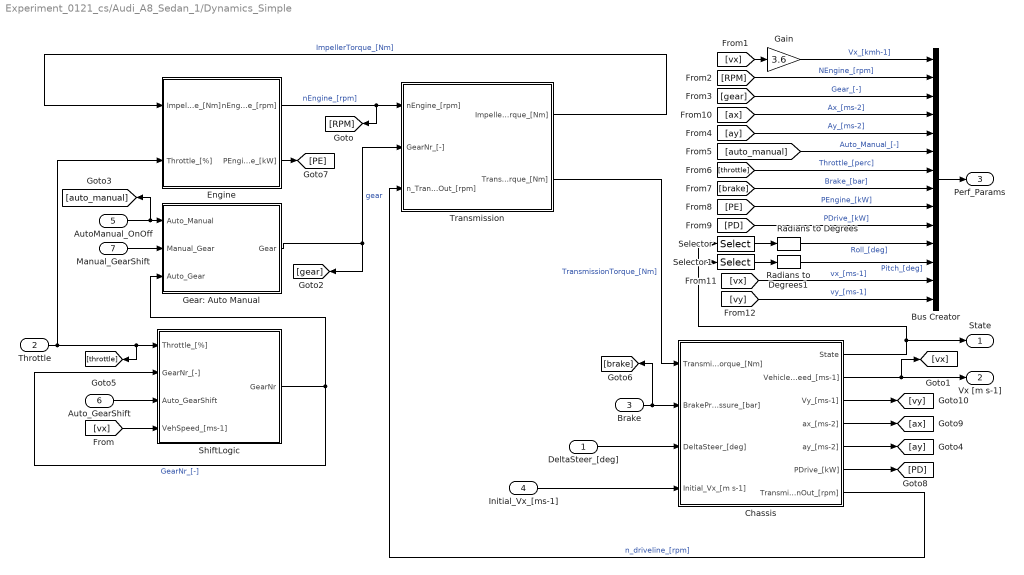
== system Experiment_0121_cs/Audi_A8_Sedan_1/Dynamics_Simple ==
  DeltaSteer_[deg] : Inport
  Throttle : Inport  Port=2
  Brake : Inport  Port=3
  Initial_Vx_[ms-1] : Inport  Port=4
  AutoManual_OnOff : Inport  Port=5
  Auto_GearShift : Inport  Port=6
  Manual_GearShift : Inport  Port=7
  Bus Creator : BusCreator  Inputs=14
  Chassis : Subsystem
      mask Display: image(imread('Chassis.png'));
  Engine : Subsystem
      mask Display: image(imread('Engine.png'));
  Gain : Gain  Gain=3.6
  Gear: Auto Manual : Subsystem
  Radians to Degrees : simulink_extras/Transformations/Radians to Degrees
  Radians to Degrees1 : simulink_extras/Transformations/Radians to Degrees
  Selector : Selector  InputPortWidth=9  IndexOptions=Index vector (dialog)  Indices=7  OutputSizes=1
  Selector1 : Selector  InputPortWidth=9  IndexOptions=Index vector (dialog)  Indices=8  OutputSizes=1
  ShiftLogic : Subsystem
      mask Display: image(imread('Gearshift.png'));
  Transmission : Subsystem
      mask Display: image(imread('Transmission.png'));
  State : Outport
  Vx [m s-1] : Outport  Port=2
  Perf_Params : Outport  Port=3
  wires:
  [vy] -> Bus Creator/14  "vy_[ms-1]"
  [vx] -> Bus Creator/13  "vx_[ms-1]"
  Chassis/7(TransmissionOut_[rpm]) -> Transmission/3(n_TransmissionOut_[rpm])  "n_driveline_[rpm]"
  Chassis/6(PDrive_[kW]) -> [PD]
  Chassis/5(ay_[ms-2]) -> [ay]
  Chassis/4(ax_[ms-2]) -> [ax]
  Chassis/3(Vy_[ms-1]) -> [vy]
  [vx] -> ShiftLogic/4(VehSpeed_[ms-1])
  Gear: Auto Manual/1(Gear) -> Transmission/2(GearNr_[-]), [gear]  "gear"
  Manual_GearShift/1 -> Gear: Auto Manual/2(Manual_Gear)
  AutoManual_OnOff/1 -> Gear: Auto Manual/1(Auto_Manual), [auto_manual]
  Chassis/2(VehicleSpeed_[ms-1]) -> [vx], Vx [m s-1]/1
  Auto_GearShift/1 -> ShiftLogic/3(Auto_GearShift)
  Throttle/1 -> Engine/2(Throttle_[%]), ShiftLogic/1(Throttle_[%]), [throttle]
  Initial_Vx_[ms-1]/1 -> Chassis/4(Initial_Vx_[m s-1])
  DeltaSteer_[deg]/1 -> Chassis/3(DeltaSteer_[deg])
  Chassis/1(State) -> State/1, Selector/1, Selector1/1
  Brake/1 -> [brake], Chassis/2(BrakePressure_[bar])
  Engine/1(nEngine_[rpm]) -> [RPM], Transmission/1(nEngine_[rpm])  "nEngine_[rpm]"
  ShiftLogic/1(GearNr) -> Gear: Auto Manual/3(Auto_Gear), ShiftLogic/2(GearNr_[-])  "GearNr_[-]"
  Transmission/2(TransmissionTorque_[Nm]) -> Chassis/1(TransmissionTorque_[Nm])  "TransmissionTorque_[Nm]"
  Transmission/1(ImpellerTorque_[Nm]) -> Engine/1(ImpellerTorque_[Nm])  "ImpellerTorque_[Nm]"
  Gain/1 -> Bus Creator/1  "Vx_[kmh-1]"
  [RPM] -> Bus Creator/2  "NEngine_[rpm]"
  [gear] -> Bus Creator/3  "Gear_[-]"
  [ay] -> Bus Creator/5  "Ay_[ms-2]"
  [auto_manual] -> Bus Creator/6  "Auto_Manual_[-]"
  [throttle] -> Bus Creator/7  "Throttle_[perc]"
  [brake] -> Bus Creator/8  "Brake_[bar]"
  Engine/2(PEngine_[kW]) -> [PE]
  Bus Creator/1 -> Perf_Params/1
  [PE] -> Bus Creator/9  "PEngine_[kW]"
  Radians to Degrees/1 -> Bus Creator/11  "Roll_[deg]"
  Radians to Degrees1/1 -> Bus Creator/12  "Pitch_[deg]"
  [PD] -> Bus Creator/10  "PDrive_[kW]"
  Selector/1 -> Radians to Degrees/1
  Selector1/1 -> Radians to Degrees1/1
  [vx] -> Gain/1
  [ax] -> Bus Creator/4  "Ax_[ms-2]"

== system Experiment_0121_cs/Audi_A8_Sedan_1/SELF_Demux ==
  SELF : Inport  OutDataTypeStr=Bus: PRESCAN_SELFSENSORDATA
  Bus Selector : BusSelector  OutputSignals=PositionX,PositionY,PositionZ,OrientationRoll,OrientationPitch,OrientationYaw,Velocity,Yaw_rate,Lat,Long,Alt
  Demux2 : Demux  Outputs=3
  Gain : Gain  Gain=180/pi
  Gain1 : Gain  Gain=180/pi
  Vector Concatenate1 : Concatenate  NumInputs=3
  compas converter : Subsystem
  x [m] : Outport
  y [m] : Outport  Port=2
  z [m] : Outport  Port=3
  rotx [deg] : Outport  Port=4
  roty [deg] : Outport  Port=5
  rotz [deg] : Outport  Port=6
  GPS lat [deg] : Outport  Port=7
  GPS long [deg] : Outport  Port=8
  GPS alt [m] : Outport  Port=9
  velocity [m/s] : Outport  Port=10
  heading [deg] : Outport  Port=11
  yaw rate [deg/s] : Outport  Port=12
  wires:
  Bus Selector/11 -> GPS alt [m]/1  "<Alt>"
  Bus Selector/10 -> GPS long [deg]/1  "<Long>"
  Bus Selector/9 -> GPS lat [deg]/1  "<Lat>"
  Bus Selector/8 -> Gain1/1  "<Yaw_rate>"
  Bus Selector/7 -> velocity [m/s]/1  "<Velocity>"
  Bus Selector/6 -> compas converter/1(rotz [rad]), Vector Concatenate1/3  "<OrientationYaw>"
  Bus Selector/5 -> Vector Concatenate1/2  "<OrientationPitch>"
  Bus Selector/4 -> Vector Concatenate1/1  "<OrientationRoll>"
  Vector Concatenate1/1 -> Gain/1
  Bus Selector/3 -> z [m]/1  "<PositionZ>"
  Bus Selector/2 -> y [m]/1  "<PositionY>"
  Bus Selector/1 -> x [m]/1  "<PositionX>"
  SELF/1 -> Bus Selector/1
  Gain/1 -> Demux2/1
  Demux2/1 -> rotx [deg]/1
  Demux2/2 -> roty [deg]/1
  Demux2/3 -> rotz [deg]/1
  compas converter/1(heading [deg]) -> heading [deg]/1
  Gain1/1 -> yaw rate [deg/s]/1

== system Experiment_0121_cs/Audi_A8_Sedan_1/STATE_Audi_A8_Sedan_1 ==
  State : Inport  SampleTime=TimeStep
  Bus Creator : BusCreator  Inputs=15  OutDataTypeStr=Bus: PRESCAN_STATEACTUATORDATA  NonVirtualBus=on
  Demux : Demux  Outputs=15
  iniBODYAngles wrtVEH [rad] : Constant  Value=[Roll0 Pitch0 0]  SampleTime=TimeStep
  iniVEHAngles wrtGLOB [rad] : Constant  Value=[0 0 Yaw0]  SampleTime=TimeStep
  iniVEHposition wrtGLOB [m] : Constant  Value=[x0 y0 z0]  SampleTime=TimeStep
  state2FullState : PreScanSimulinkLibrary/state2FullState  SystemSampleTime=-1
  StateBus : Outport  OutDataTypeStr=Bus: PRESCAN_STATEACTUATORDATA
  wires:
  Bus Creator/1 -> StateBus/1
  State/1 -> state2FullState/1
  state2FullState/1 -> Demux/1
  iniVEHposition wrtGLOB [m]/1 -> state2FullState/2
  iniBODYAngles wrtVEH [rad]/1 -> state2FullState/3
  iniVEHAngles wrtGLOB [rad]/1 -> state2FullState/4
  Demux/1 -> Bus Creator/1  "PositionX"
  Demux/2 -> Bus Creator/2  "PositionY"
  Demux/3 -> Bus Creator/3  "PositionZ"
  Demux/4 -> Bus Creator/4  "VelocityX"
  Demux/5 -> Bus Creator/5  "VelocityY"
  Demux/6 -> Bus Creator/6  "VelocityZ"
  Demux/7 -> Bus Creator/7  "AccelerationX"
  Demux/8 -> Bus Creator/8  "AccelerationY"
  Demux/9 -> Bus Creator/9  "AccelerationZ"
  Demux/10 -> Bus Creator/10  "OrientationRoll"
  Demux/11 -> Bus Creator/11  "OrientationPitch"
  Demux/12 -> Bus Creator/12  "OrientationYaw"
  Demux/13 -> Bus Creator/13  "AngularVelocityRoll"
  Demux/14 -> Bus Creator/14  "AngularVelocityPitch"
  Demux/15 -> Bus Creator/15  "AngularVelocityYaw"

== system Experiment_0121_cs/Audi_A8_Sedan_1/Trajectories ==
  Traj2State1 : Subsystem  Tag=Traj2State  mask(PreScan Demux Block:){}
      settings: DeleteFcn=PreScanBlockDeleteFcn;
  TrajCoGOffset : Subsystem  Tag=TrajCoGOffset  mask(Trajectory CoG Offset block){CoGOffsetZ=0.55, InitRoll=0, InitPitch=0}
      mask prompts: CoGOffsetZ "Z-component of CoG Offset [m]:"; InitRoll "Initial Roll angle [deg]:"; InitPitch "Initial Pitch angle [deg]:"
      mask help: A trajectory follows the surface of the road. However the position of a actor is based on the actor's Center of Gravity, which is typically above the road. This block converts from the trajectory along the road surface to the trajectory of the actor's CoG by realigning the z-component of the CoG offset to be normal to the road.
      settings: DeleteFcn=PreScanBlockDeleteFcn;
  Trajectory_1 : Subsystem  Tag=Trajectory  mask(PreScan Source Block: Trajectory){FileName='Trajectory_1.mat', TimeStep=1/20}
      mask prompts: TimeStep "Time Step [s]"
      mask help:
      | The Trajectory block contains the trajectories defined in the PreScan Experiment Editor. The output of the trajectory block is the (vehicle) State.
      |
      | For more information, please click Help.
      mask init:
      | EXPROOT=pwd;  % TODO better construction for locating base experiment
      | 
      | trajfilename = fullfile(EXPROOT,'Trajectories',FileName);
      | load(trajfilename);
      | trajectory=trajectory';
      | 
      | traj.time=trajectory(:,1);%[];
      | traj.signals.values=trajectory(:,2:19);
      | traj.dimensions=18;
      | traj.label='';
      | 
      | SampleTime=traj.time(2)-traj.time(1);
      settings: DeleteFcn=PreScanBlockDeleteFcn;
      mask Help: eval('openHelp(312)')
      mask Display: fprintf(FileName)
  Trajectory_1_Offset : Constant  Tag=TrajectoryOffset  Value="[0  0  0  0  0  0]"
  State : Outport  Tag=TrajOutport
  wires:
  Trajectory_1/1(trajectory) -> Traj2State1/1(Traj Org)
  Trajectory_1_Offset/1 -> Traj2State1/2(Offset)
  TrajCoGOffset/1(State Out) -> State/1
  Traj2State1/1(state) -> TrajCoGOffset/1(State In)
